simulink model "PID_notcomp"  (R2024b)
settings: Solver=VariableStepAuto  StartTime=0.0  StopTime=9  RelTol=1e-5
model workspace (MATLAB code in the model file):
  | %liqud data
  | rho_l = 850;
  | 
  | %valve data
  | pRat = 30e5; %rated pressure
  | Cd = 0.6; %discarge coefficient
  | QRat = 270/6e4;
  | Admax = QRat/Cd/(2/rho_l*pRat/2)^0.5;
  | 
  | %Cylinder 1
  | sC_1 = 0.45; %Stroke
  | L0C_1 = 0.4; %Deadlength
  | x0C_1 = 0.2; %Initial position
  | dC_1 = 0.065; %Piston diameter
  | dRC_1 = 0.035; %Rod diameter
  | %Derived values
  | dOC_1 = dC_1 + dC_1/4; %Cylinder outer diameter
  | LC_1 = sC_1 + L0C_1/3; %Cylinder length
  | tEPC_1 = L0C_1/6; %Thickness of end plate
  | dJC_1 = L0C_1/3; %Diameter of joint
  | LJC_1 = dRC_1; %Length of joint
  | LRC_1 = sC_1 + tEPC_1; %Length of rod
  | tPC_1 = L0C_1/3; %Thickness of piston
  | AC_1 = pi*dC_1^2/4; %Piston area
  | ARC_1 = pi*dRC_1^2/4; %Rod area
  | AAC_1 = AC_1 - ARC_1; %Annulus area
  | 
  | % crane arm
  | g=9.81;
  | theta1_init=0*pi/180;
  | thetaDot1_init=0;
  | L1=3.625;
  | rho=7800;
  | L4 = 0.229;
  | Lg4x = L1-L4/2;
  | Lg4y = 0.08157;
  | 
  | % initial cylinder position
  | Cy = -1.055;
  | Cx = 0.420;
  | abx = 0.550;
  | aby = -0.130;
undefined symbols (not defined in the file): X, Y, Z
libraries: sm_lib x35, fl_lib x22, nesl_utility x18, SimscapeFluids_lib x6, slpidlib x1
(part 3 of 3)

== matlab function PID_notcomp/Subsystem/MATLAB Function ==
  data: u input; pLS output; pA input; pB input
function pLS = fcn(u,pA,pB)
uEps = 0.05; %Deadband
if u < -uEps
    pLS = pB;
elseif u < uEps
    pLS = 0;
else
    pLS = pA;
end

== matlab function PID_notcomp/CTRL/MATLAB Function ==
  data: u_ref input; U output
function U = fcn(u_ref)
BW = 0.8; % Bandwidth
SpoolTravel = 7; % Maximum Spool Travel
if u_ref >0
    U = u_ref+BW/SpoolTravel;
elseif u_ref < 0
     U = u_ref-BW/SpoolTravel;
else 
     U = 0;
end
